simulink model "kidneyy"  (R2022a)
settings: Solver=VariableStepAuto  StartTime=0.0  StopTime=10.0  RelTol=1e-3
libraries: simulink x5
settings Model: Creator=Dell  LastModifiedBy=Dell

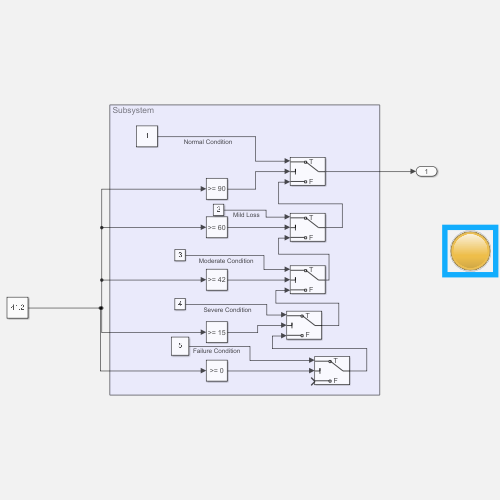
[thumbnail: Simulink's stored preview of the top-level diagram]
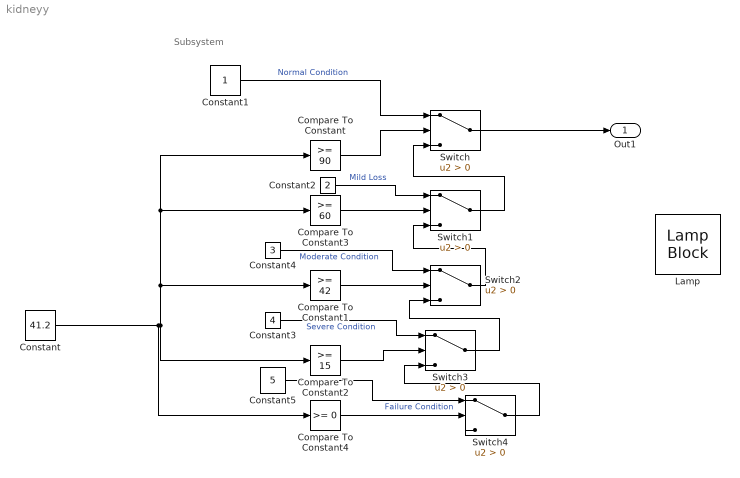
== system kidneyy ==
  note: Subsystem
  Compare To Constant : simulink/Logic and Bit Operations/Compare To Constant  relop=>=  const=90  OutDataTypeStr=boolean
  Compare To Constant1 : simulink/Logic and Bit Operations/Compare To Constant  relop=>=  const=42  OutDataTypeStr=boolean
  Compare To Constant2 : simulink/Logic and Bit Operations/Compare To Constant  relop=>=  const=15  OutDataTypeStr=boolean
  Compare To Constant3 : simulink/Logic and Bit Operations/Compare To Constant  relop=>=  const=60  OutDataTypeStr=boolean
  Compare To Constant4 : simulink/Logic and Bit Operations/Compare To Constant  relop=>=  const=0  OutDataTypeStr=boolean
  Constant : Constant  Value=41.2
  Constant1 : Constant
  Constant2 : Constant  Value=2
  Constant3 : Constant  Value=4
  Constant4 : Constant  Value=3
  Constant5 : Constant  Value=5
  Lamp : LampBlock  LabelPosition=Hide
  Switch{,1..4} (5 alike) : Switch  Criteria=u2 > Threshold  SaturateOnIntegerOverflow=off  InputSameDT=off
  Out1 : Outport
  wires:
  Constant5/1 -> Switch4/1  "Failure Condition"
  Switch4/1 -> Switch3/3
  Compare To Constant4/1 -> Switch4/2
  Compare To Constant1/1 -> Switch2/2
  Compare To Constant2/1 -> Switch3/2
  Constant2/1 -> Switch1/1  "Mild Loss"
  Switch3/1 -> Switch2/3
  Constant1/1 -> Switch/1  "Normal Condition"
  Constant3/1 -> Switch3/1  "Severe Condition"
  Compare To Constant3/1 -> Switch1/2
  Constant4/1 -> Switch2/1  "Moderate Condition"
  Switch2/1 -> Switch1/3
  Switch1/1 -> Switch/3
  Constant/1 -> Compare To Constant3/1, Compare To Constant/1, Compare To Constant1/1, Compare To Constant2/1, Compare To Constant4/1
  Compare To Constant/1 -> Switch/2
  Switch/1 -> Out1/1
